simulink model "iron"  (R2020b)
settings: Solver=ode4  StartTime=0.0  StopTime=t  FixedStep=0.1  RelTol=1e-3
values from neighbouring files (symbols this model uses):
  A = 0.05    [init_iron.m]
  alpha = 15    [init_iron.m]
  cp = 449    [init_iron.m]
  m = 0.5    [init_iron.m]
  PB = 1000    [init_iron.m]
  Tamb = 20    [init_iron.m]
  Tdes = 100    [init_iron.m]
  Tdiff = 10    [init_iron.m]
settings Model: Creator=root  LastModifiedBy=root

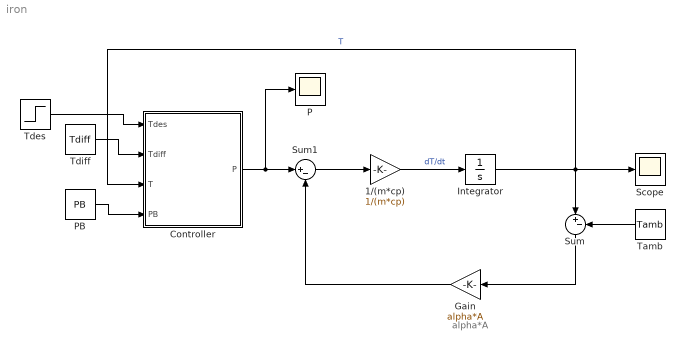
== system iron ==
  note: alpha*A
  1/(m*cp) : Gain  Gain=1/(m*cp)
  Controller : Stateflow chart  TreatAsAtomicUnit=on
  Gain : Gain  Gain=alpha*A
  Integrator : Integrator  InitialCondition=Tamb
  P : Scope
  PB : Constant  Value=PB
  Scope : Scope
  Sum : Sum  Inputs=|+-
  Sum1 : Sum  Inputs=|+-
  Tamb : Constant  Value=Tamb
  Tdes : Step  Time=0  After=Tdes  SampleTime=0
  Tdiff : Constant  Value=Tdiff
  wires:
  1/(m*cp)/1 -> Integrator/1  "dT/dt"
  Integrator/1 -> Controller/3(T), Sum/1, Scope/1  "T"
  Tamb/1 -> Sum/2
  Sum/1 -> Gain/1
  Gain/1 -> Sum1/2
  Sum1/1 -> 1/(m*cp)/1
  Tdes/1 -> Controller/1(Tdes)
  Tdiff/1 -> Controller/2(Tdiff)
  Controller/1(P) -> P/1, Sum1/1
  PB/1 -> Controller/4(PB)

== stateflow chart iron/Controller ==
  state CLOSED
    P=PB;
  state OPEN
    P=0;
  CLOSED -> OPEN : [T > Tdes ]
  OPEN -> CLOSED : [T<Tdes-Tdiff]
  (default) -> OPEN
  data: Tdes input; Tdiff input; T input; P output; PB input
